simulink model "Single_Pendulum_balance"  (R2021a)
settings: Solver=ode4  StartTime=0.0  StopTime=50  FixedStep=0.001  RelTol=1e-3
undefined symbols (not defined in the file): sp_control_vector, sp_dynamics_vector
settings Model: Creator=YW  LastModifiedBy=YW

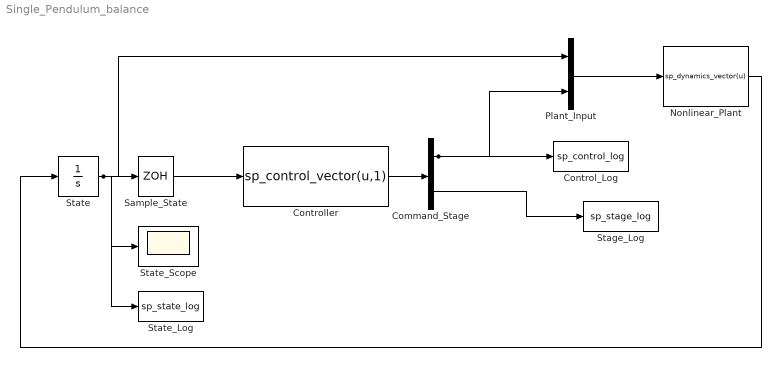
== system Single_Pendulum_balance ==
  Command_Stage : Demux  Outputs=2
  Control_Log : ToWorkspace  VariableName=sp_control_log  SaveFormat=Structure With Time  SampleTime=-1
  Controller : MATLABFcn  MATLABFcn=sp_control_vector(u,1)  OutputDimensions=2
  Nonlinear_Plant : MATLABFcn  MATLABFcn=sp_dynamics_vector(u)  OutputDimensions=4
  Plant_Input : Mux  Inputs=2
  Sample_State : ZeroOrderHold  SampleTime=0.001
  Stage_Log : ToWorkspace  VariableName=sp_stage_log  SaveFormat=Structure With Time  SampleTime=-1
  State : Integrator  InitialCondition=[0;0.10000000000000001;0;0]
  State_Log : ToWorkspace  VariableName=sp_state_log  SaveFormat=Structure With Time  SampleTime=-1
  State_Scope : Scope
  wires:
  Command_Stage/1 -> Plant_Input/2, Control_Log/1
  Command_Stage/2 -> Stage_Log/1
  Plant_Input/1 -> Nonlinear_Plant/1
  Nonlinear_Plant/1 -> State/1
  Controller/1 -> Command_Stage/1
  Sample_State/1 -> Controller/1
  State/1 -> Sample_State/1, Plant_Input/1, State_Log/1, State_Scope/1
